simulink model "Good_1PF_Template_Copy"  (R2022b)
settings: Solver=FixedStepAuto  StartTime=0.0  StopTime=30  FixedStep=0.10  RelTol=1e-3
undefined symbols (not defined in the file): D1, D2, estimated_W_xu, initial_guess_belief_car2, num_particles, std_dev, W_xu_ranges, x0
settings Model: Creator=user  LastModifiedBy=user

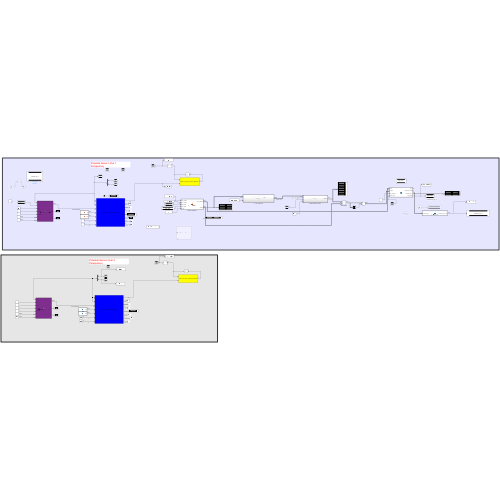
[thumbnail: Simulink's stored preview of the top-level diagram]
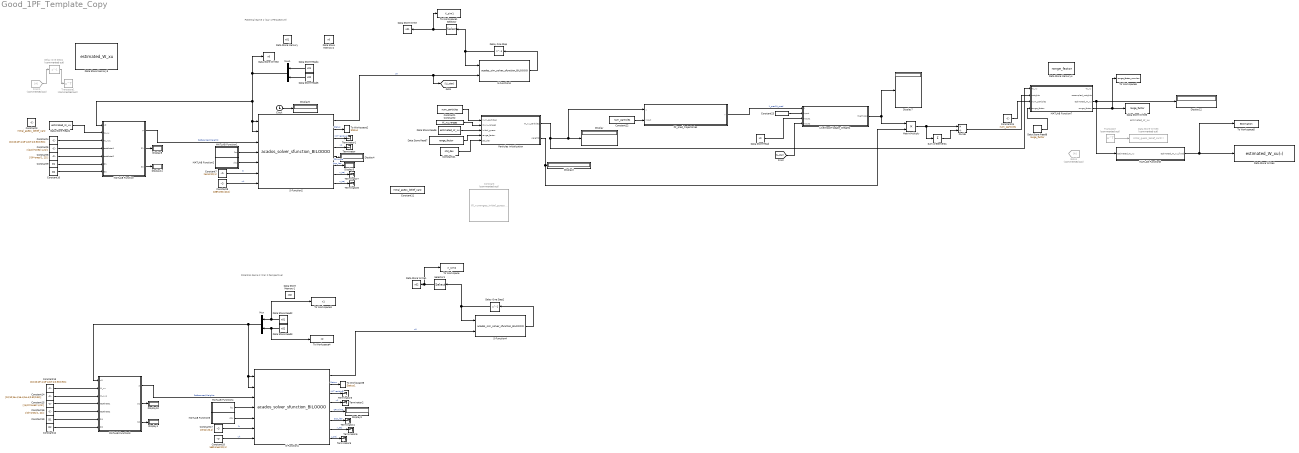
== system Good_1PF_Template_Copy ==
  note: estimated_W_xu
  note: Potential Game 1 (Car 1 Perspective)
  note: Potential Game 2 (Car 2 Perspective)
  Clock : Clock
  Constant : Constant  Commented=on  Value=W_xuranges_initial_guess...
  Constant{1,22..24} (4 alike) : Constant  Value=num_particles
  Constant10 : Constant  Value=D2
  Constant11 : Constant  Value=initial_guess_belief_car2
  Constant12 : Constant  Value=D2
  Constant13 : Constant  Value=[10;10;1e-4;1e-4;1e-4;0.50;0.50];
  Constant14 : Constant  Value=[10;10;1e-4;1e-4;1e-4;0.50;0.50];
  Constant15 : Constant  Value=[(pi/2)*ones(1,21)]
  Constant16 : Constant  Value=[(0)*ones(1, 21)]
  Constant17 : Constant  Value=zeros(20,1)
  Constant18 : Constant  Value=1e8*ones(20,1)
  Constant19 : Constant  Value=D1
  Constant2 : Constant  Value=W_xu_ranges
  Constant21 : Constant  Value=std_dev
  Constant3 : Constant  Value=initial_guess_belief_car2
  Constant4 : Constant  Value=[10;10;1e-4;1e-4;1e-4;0.50;0.50];
  Constant5 : Constant  Value=[(pi/2)*ones(1,21)]
  Constant6 : Constant  Value=[(0)*ones(1, 21)]
  Constant7 : Constant  Value=zeros(20,1)
  Constant8 : Constant  Value=1e8*ones(20,1)
  Constant9 : Constant  Value=D1
  Data Store Memory : DataStoreMemory  DataStoreName=x01  WriteAfterWriteMsg=warning  InitialValue=x01  ShowAdditionalParam=off
  Data Store Memory1 : DataStoreMemory  DataStoreName=x02  WriteAfterWriteMsg=warning  InitialValue=x02  ShowAdditionalParam=off
  Data Store Memory2 : DataStoreMemory  DataStoreName=x0  WriteAfterWriteMsg=warning  InitialValue=x0  ShareAcrossModelInstances=on  ShowAdditionalParam=off
  Data Store Memory3 : DataStoreMemory  DataStoreName=estimated_W_xu  WriteAfterWriteMsg=warning  InitialValue=initial_guess_belief_car2  ShowAdditionalParam=off
  Data Store Memory4 : DataStoreMemory  DataStoreName=range_factor  WriteAfterWriteMsg=warning  InitialValue=1  ShowAdditionalParam=off
  Data Store Read : DataStoreRead  DataStoreName=x0  IndexOptions=Index vector (dialog)  Indices=1  OutputSizes=1
  Data Store Read1 : DataStoreRead  DataStoreName=estimated_W_xu  IndexOptions=Index vector (dialog)  Indices=1  OutputSizes=1
  Data Store Read2 : DataStoreRead  DataStoreName=x01  IndexOptions=Index vector (dialog)  Indices=1  OutputSizes=1
  Data Store Read3 : DataStoreRead  DataStoreName=x02  IndexOptions=Index vector (dialog)  Indices=1  OutputSizes=1
  Data Store Read4 : DataStoreRead  DataStoreName=x01  IndexOptions=Index vector (dialog)  Indices=1  OutputSizes=1
  Data Store Read5 : DataStoreRead  DataStoreName=x02  IndexOptions=Index vector (dialog)  Indices=1  OutputSizes=1
  Data Store Read6 : DataStoreRead  DataStoreName=estimated_W_xu  IndexOptions=Index vector (dialog)  Indices=1  OutputSizes=1
  Data Store Read7 : DataStoreRead  DataStoreName=range_factor  IndexOptions=Index vector (dialog)  Indices=1  OutputSizes=1
  Data Store Read8 : DataStoreRead  DataStoreName=range_factor  IndexOptions=Index vector (dialog)  Indices=1  OutputSizes=1
  Data Store Write : DataStoreWrite  DataStoreName=x01  DataStoreElements=x01  IndexOptions=Index vector (dialog)  Indices=1  OutputSizes=1
  Data Store Write1 : DataStoreWrite  DataStoreName=x02  IndexOptions=Index vector (dialog)  Indices=1  OutputSizes=1
  Data Store Write2 : DataStoreWrite  DataStoreName=x0  IndexOptions=Index vector (dialog)  Indices=1  OutputSizes=1
  Data Store Write3 : DataStoreWrite  Commented=on  DataStoreName=initial_guess_belief_car2  DataStoreElements=initial_guess_belief_car2(:)  IndexOptions=Index vector (dialog)  Indices=1  OutputSizes=1
  Data Store Write4 : DataStoreWrite  DataStoreName=estimated_W_xu  DataStoreElements=estimated_W_xu(:)  IndexOptions=Index vector (dialog)  Indices=1  OutputSizes=1
  Data Store Write5 : DataStoreWrite  DataStoreName=range_factor  IndexOptions=Index vector (dialog)  Indices=1  OutputSizes=1
  Delay One Step : Delay  DelayLength=1  InitialCondition=x0
  Delay One Step1 : Delay  Commented=on  DelayLength=1  InitialCondition=initial_guess_belief_car2'
  Delay One Step2 : Delay  DelayLength=1  InitialCondition=x0
  Display{,1..8,10..12} (12 alike) : Display
  Divide : Product  Inputs=*/
  From1 : From  Commented=on
  Goto1 : Goto  Commented=on
  Likelihood+Ipdate_Weights : Subsystem  TreatAsAtomicUnit=on
  MATLAB Function : MATLAB Function  TreatAsAtomicUnit=on
  MATLAB Function1 : MATLAB Function  TreatAsAtomicUnit=on
  MATLAB Function2 : MATLAB Function  TreatAsAtomicUnit=on
  MATLAB Function3 : MATLAB Function  TreatAsAtomicUnit=on
  MATLAB Function4 : MATLAB Function  TreatAsAtomicUnit=on
  MATLAB Function5 : MATLAB Function  TreatAsAtomicUnit=on
  MATLAB Function7 : MATLAB Function  TreatAsAtomicUnit=on
  MATLAB Function8 : MATLAB Function  TreatAsAtomicUnit=on
  MatrixMultiply : Product
  Mux : Mux  Inputs=2
  Mux1 : Mux  Inputs=2
  PF_pred_trajectories : Subsystem  TreatAsAtomicUnit=on
  Particles initialization : MATLAB Function  TreatAsAtomicUnit=on
  S-Function1 : S-Function  FunctionName=acados_solver_sfunction_BILOOOO  SFunctionDeploymentMode=off  EnableBusSupport=off
  S-Function2 : S-Function  FunctionName=acados_solver_sfunction_BILOOOO  SFunctionDeploymentMode=off  EnableBusSupport=off
  S-Function3 : S-Function  FunctionName=acados_sim_solver_sfunction_BILOOOO  SFunctionDeploymentMode=off  EnableBusSupport=off
  S-Function4 : S-Function  FunctionName=acados_sim_solver_sfunction_BILOOOO  SFunctionDeploymentMode=off  EnableBusSupport=off
  Selector : Selector  InputPortWidth=10  IndexOptions=Index vector (dialog)  Indices=[1:5]  OutputSizes=1
  Selector1 : Selector  InputPortWidth=10  IndexOptions=Index vector (dialog)  Indices=[6:10]  OutputSizes=1
  Sum of Elements : Sum  Inputs=+
  Terminator{,1..8} (9 alike) : Terminator
  To Workspace : ToWorkspace  VariableName=X_sim2  SaveFormat=Structure With Time  SampleTime=-1
  To Workspace1 : ToWorkspace  VariableName=X_sim1  SaveFormat=Structure With Time  SampleTime=-1
  To Workspace2 : ToWorkspace  VariableName=Status  SampleTime=-1
      settings: Save2DSignal=2-D array (concatenate along first dimension)
  To Workspace3 : ToWorkspace  VariableName=x1  SaveFormat=Structure  SampleTime=-1
  To Workspace4 : ToWorkspace  VariableName=x2  SaveFormat=Structure  SampleTime=-1
  To Workspace5 : ToWorkspace  VariableName=Estimation  SampleTime=-1
      settings: Save2DSignal=2-D array (concatenate along first dimension)
  To Workspace6 : ToWorkspace  VariableName=range_factor_monitor  SampleTime=-1
      settings: Save2DSignal=2-D array (concatenate along first dimension)
  To Workspace8 : ToWorkspace  VariableName=Status1  SampleTime=-1
      settings: Save2DSignal=2-D array (concatenate along first dimension)
  Transpose : Math  Commented=on  Operator=transpose
  Transpose1 : Math  Commented=on  Operator=transpose
  wires:
  Constant14/1 -> MATLAB Function3/3(W_xu1)
  Mux1/1 -> Data Store Write2/1, S-Function2/2, S-Function2/1, MATLAB Function/1(x0)
  Data Store Read5/1 -> Mux1/2
  S-Function4/1 -> Delay One Step2/1
  Constant19/1 -> MATLAB Function3/6(D1)
  Constant15/1 -> MATLAB Function3/4(testtheta1)
  Constant7/1 -> S-Function2/6  "lh"
  MATLAB Function1/1(lbu) -> S-Function2/4
  MATLAB Function/2(S1) -> Display8/1
  MATLAB Function/1(p) -> S-Function2/3  "References|Weights"
  S-Function2/4 -> Terminator/1  "x1"
  Data Store Read3/1 -> To Workspace4/1, Mux/2
  MATLAB Function3/3(S2) -> Display1/1
  S-Function1/7 -> Terminator6/1  "x_traj"
  S-Function2/3 -> Terminator1/1  "KKT residual"
  MATLAB Function4/1(lbu) -> S-Function1/4
  Delay One Step/1 -> Selector/1, S-Function3/1
  Constant13/1 -> MATLAB Function3/2(W_xu)
  Constant17/1 -> S-Function1/6  "lh"
  S-Function3/1 -> Delay One Step/1
  Constant8/1 -> S-Function2/7  "uh"
  MATLAB Function/3(S2) -> Display11/1
  Delay One Step2/1 -> Selector1/1, S-Function4/1
  S-Function2/2 -> To Workspace2/1  "Status"
  S-Function1/2 -> To Workspace8/1  "Status"
  MATLAB Function3/1(p) -> S-Function1/3  "References|Weights"
  MATLAB Function5/1(ubu) -> S-Function1/5
  S-Function1/3 -> Terminator3/1  "KKT residual"
  Clock/1 -> Display6/1
  Constant10/1 -> MATLAB Function/7(D2)
  S-Function2/8 -> Terminator8/1  "u_traj"
  S-Function1/5 -> Display3/1  "CPU time"
  S-Function1/4 -> Terminator2/1  "x1"
  Constant4/1 -> MATLAB Function/3(W_xu1)
  Constant16/1 -> MATLAB Function3/5(testtheta2)
  MATLAB Function2/1(ubu) -> S-Function2/5
  Mux/1 -> S-Function1/2, S-Function1/1, MATLAB Function3/1(x0)
  Data Store Read4/1 -> Mux1/1
  S-Function1/6 -> Terminator4/1  "Sqp_iter"
  Constant6/1 -> MATLAB Function/5(testtheta2)
  S-Function1/1 -> S-Function4/2  "u0"
  S-Function2/6 -> Display5/1  "Sqp_iter"
  S-Function2/1 -> [U_star], S-Function3/2  "u0"
  MATLAB Function3/2(S1) -> Display10/1
  S-Function1/8 -> Terminator5/1  "u_traj"
  Constant5/1 -> MATLAB Function/4(testtheta1)
  Selector/1 -> To Workspace1/1, Data Store Write/1
  Selector1/1 -> To Workspace/1, Data Store Write1/1
  S-Function2/5 -> Display4/1  "CPU time"
  Constant9/1 -> MATLAB Function/6(D1)
  S-Function2/7 -> Terminator7/1  "x_traj"
  Data Store Read2/1 -> To Workspace3/1, Mux/1
  Constant12/1 -> MATLAB Function3/7(D2)
  Constant18/1 -> S-Function1/7  "uh"
  Constant1/1 -> Particles initialization/1(num_particles)
  Data Store Read7/1 -> Particles initialization/4(range_factor)
  Constant2/1 -> Particles initialization/2(W_xu_ranges)
  Constant21/1 -> Particles initialization/5(std_dev)
  Particles initialization/1(W_xu_particles) -> PF_pred_trajectories/1(y), Display/1, MATLAB Function7/1("W_xu ")
  Particles initialization/2(weights) -> MatrixMultiply/2, Display2/1
  Constant22/1 -> PF_pred_trajectories/2(Input)
  PF_pred_trajectories/1(Y) -> Likelihood+Ipdate_Weights/1(Y)  "X_pred|U_pred"
  Constant23/1 -> Likelihood+Ipdate_Weights/2(Input)
  Data Store Read/1 -> Likelihood+Ipdate_Weights/3(Input1)
  [U_star] -> Likelihood+Ipdate_Weights/4(Input2)
  Likelihood+Ipdate_Weights/1(likelihood) -> MatrixMultiply/1, Display7/1
  MatrixMultiply/1 -> Sum of Elements/1, Divide/1
  Sum of Elements/1 -> Divide/2
  Divide/1 -> MATLAB Function7/2(weights)
  Constant24/1 -> MATLAB Function7/3(num_particles)
  MATLAB Function7/3(estimated_W_xu) -> MATLAB Function8/1(estimated_W_xu), Display12/1
  Transpose/1 -> Data Store Write3/1
  From1/1 -> Delay One Step1/1
  Delay One Step1/1 -> Transpose1/1
  Data Store Read1/1 -> MATLAB Function/2(W_xu)
  MATLAB Function8/1(estimated_W_xu_fixed) -> To Workspace5/1, Data Store Write4/1
  Data Store Read6/1 -> Particles initialization/3(initial_guess)
  MATLAB Function7/4(range_factor) -> To Workspace6/1, Data Store Write5/1
  Data Store Read8/1 -> MATLAB Function7/4("range_factor ")

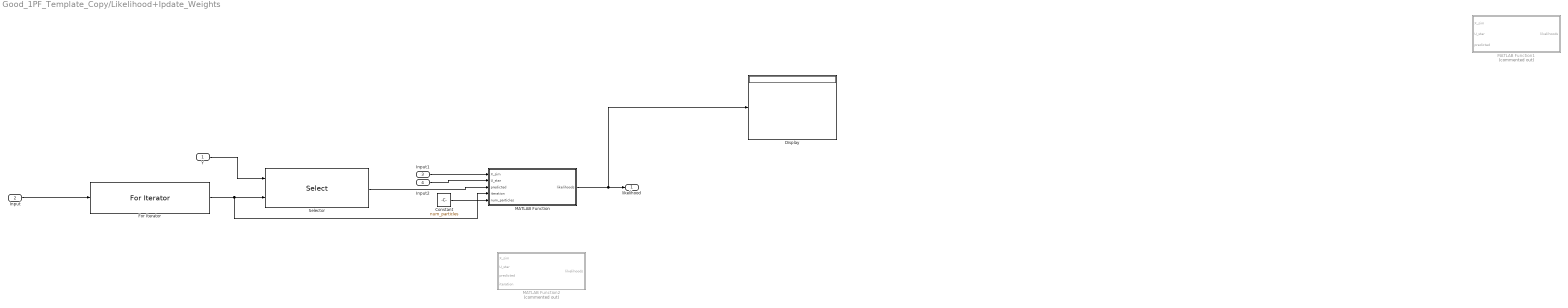
== system Good_1PF_Template_Copy/Likelihood+Ipdate_Weights ==
  Y : Inport
  Input : Inport  Port=2
  Input1 : Inport  Port=3
  Input2 : Inport  Port=4
  Constant : Constant  Value=num_particles
  Display : Display
  For Iterator : ForIterator  IterationSource=external
  MATLAB Function : MATLAB Function  TreatAsAtomicUnit=on
  MATLAB Function1 : MATLAB Function  Commented=on  TreatAsAtomicUnit=on
  MATLAB Function2 : MATLAB Function  Commented=on  TreatAsAtomicUnit=on
  Selector : Selector  NumberOfDimensions=2  IndexOptions=Select all,Index vector (port)  Indices=[1 3],1  OutputSizes=1,1  RuntimeRangeChecks=on
  likelihood : Outport
  wires:
  Input/1 -> For Iterator/1
  For Iterator/1 -> MATLAB Function/4(iteration), Selector/2
  Y/1 -> Selector/1
  Selector/1 -> MATLAB Function/3(predicted)
  Input1/1 -> MATLAB Function/1(X_sim)
  Input2/1 -> MATLAB Function/2(U_star)
  MATLAB Function/1(likelihoods) -> Display/1, likelihood/1
  Constant/1 -> MATLAB Function/5(num_particles)

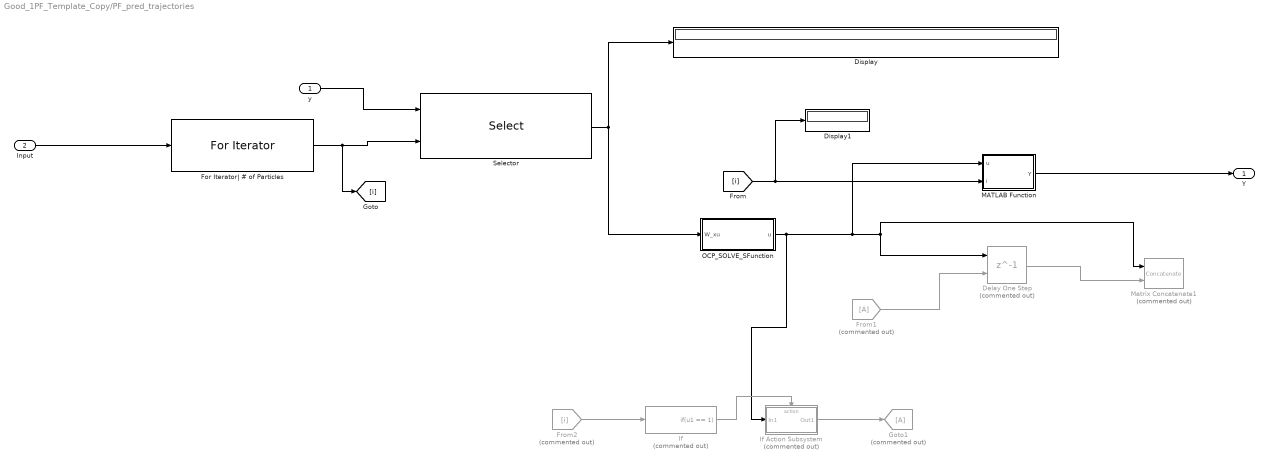
== system Good_1PF_Template_Copy/PF_pred_trajectories ==
  y : Inport
  Input : Inport  Port=2
  Delay One Step : Delay  Commented=on  DelayLength=1  InitialConditionSource=Input port
      settings: InputPortMap=u0,p4
  Display : Display
  Display1 : Display
  For Iterator| # of Particles : ForIterator  IterationSource=external  IterationLimit=num_particles
  From1 : From  Commented=on
  From2 : From  Commented=on  GotoTag=i
  Goto1 : Goto  Commented=on
  If : If  Commented=on  IfExpression=u1 == 1  ShowElse=off
  If Action Subsystem : Subsystem  Commented=on  TreatAsAtomicUnit=on
  MATLAB Function : MATLAB Function  TreatAsAtomicUnit=on
  Matrix Concatenate1 : Concatenate  Commented=on  Mode=Multidimensional array  ConcatenateDimension=2
  OCP_SOLVE_SFunction : Subsystem
  Selector : Selector  NumberOfDimensions=2  IndexOptions=Index vector (port),Select all  Indices=[1 3],1  OutputSizes=1,1  RuntimeRangeChecks=on
  Y : Outport
  wires:
  Input/1 -> For Iterator| # of Particles/1
  For Iterator| # of Particles/1 -> [i], Selector/2
  y/1 -> Selector/1
  Selector/1 -> OCP_SOLVE_SFunction/1(W_xu), Display/1
  OCP_SOLVE_SFunction/1(u) -> MATLAB Function/1(u), Delay One Step/1, Matrix Concatenate1/1, If Action Subsystem/1(In1)
  If Action Subsystem/1(Out1) -> Goto1/1
  From1/1 -> Delay One Step/2
  Delay One Step/1 -> Matrix Concatenate1/2
  From2/1 -> If/1
  If/1 -> If Action Subsystem/Action
  [i] -> Display1/1, MATLAB Function/2(i)
  MATLAB Function/1(Y) -> Y/1

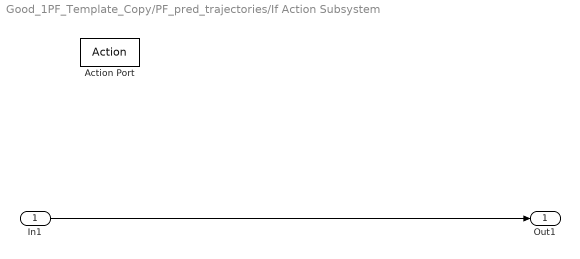
== system Good_1PF_Template_Copy/PF_pred_trajectories/If Action Subsystem ==
  In1 : Inport
  Action Port : ActionPort  ActionPortLabel=if(u1 == 1)
  Out1 : Outport
  wires:
  In1/1 -> Out1/1

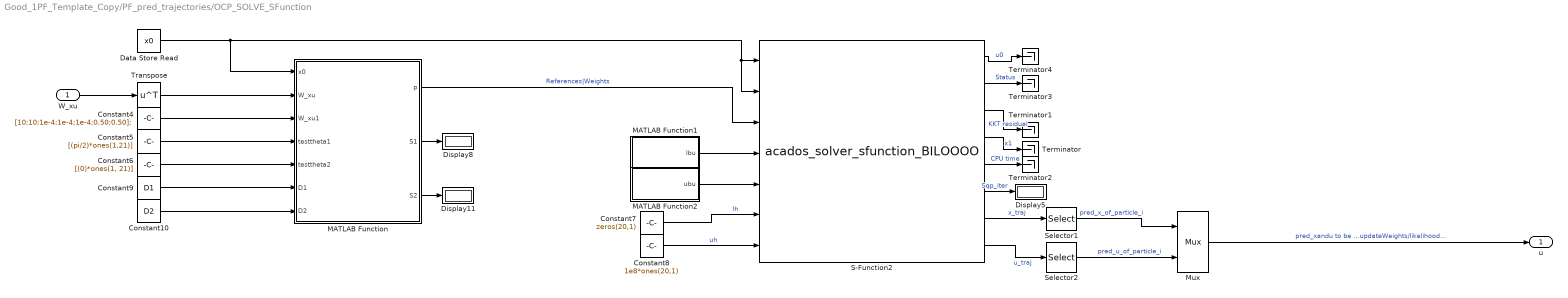
== system Good_1PF_Template_Copy/PF_pred_trajectories/OCP_SOLVE_SFunction ==
  W_xu : Inport
  Constant10 : Constant  Value=D2
  Constant4 : Constant  Value=[10;10;1e-4;1e-4;1e-4;0.50;0.50];
  Constant5 : Constant  Value=[(pi/2)*ones(1,21)]
  Constant6 : Constant  Value=[(0)*ones(1, 21)]
  Constant7 : Constant  Value=zeros(20,1)
  Constant8 : Constant  Value=1e8*ones(20,1)
  Constant9 : Constant  Value=D1
  Data Store Read : DataStoreRead  DataStoreName=x0  IndexOptions=Index vector (dialog)  Indices=1  OutputSizes=1
  Display11 : Display
  Display5 : Display
  Display8 : Display
  MATLAB Function : MATLAB Function  TreatAsAtomicUnit=on
  MATLAB Function1 : MATLAB Function  TreatAsAtomicUnit=on
  MATLAB Function2 : MATLAB Function  TreatAsAtomicUnit=on
  Mux : Mux  Inputs=2
  S-Function2 : S-Function  FunctionName=acados_solver_sfunction_BILOOOO  SFunctionDeploymentMode=off  EnableBusSupport=off
  Selector1 : Selector  InputPortWidth=210  IndexOptions=Index vector (dialog)  Indices=[11:20]  OutputSizes=1
  Selector2 : Selector  InputPortWidth=80  IndexOptions=Index vector (dialog)  Indices=[1:4]  OutputSizes=1
  Terminator{,1..4} (5 alike) : Terminator
  Transpose : Math  Operator=transpose
  u : Outport
  wires:
  MATLAB Function1/1(lbu) -> S-Function2/4
  Data Store Read/1 -> S-Function2/2, S-Function2/1, MATLAB Function/1(x0)
  S-Function2/3 -> Terminator1/1  "KKT residual"
  Constant6/1 -> MATLAB Function/5(testtheta2)
  MATLAB Function/2(S1) -> Display8/1
  S-Function2/7 -> Selector1/1  "x_traj"
  Constant4/1 -> MATLAB Function/3(W_xu1)
  MATLAB Function/1(p) -> S-Function2/3  "References|Weights"
  S-Function2/6 -> Display5/1  "Sqp_iter"
  MATLAB Function2/1(ubu) -> S-Function2/5
  Constant8/1 -> S-Function2/7  "uh"
  S-Function2/5 -> Terminator2/1  "CPU time"
  Constant5/1 -> MATLAB Function/4(testtheta1)
  MATLAB Function/3(S2) -> Display11/1
  Constant9/1 -> MATLAB Function/6(D1)
  S-Function2/4 -> Terminator/1  "x1"
  S-Function2/2 -> Terminator3/1  "Status"
  Constant10/1 -> MATLAB Function/7(D2)
  S-Function2/8 -> Selector2/1  "u_traj"
  Constant7/1 -> S-Function2/6  "lh"
  S-Function2/1 -> Terminator4/1  "u0"
  Selector1/1 -> Mux/1  "pred_x_of_particle_i"
  Selector2/1 -> Mux/2  "pred_u_of_particle_i"
  Mux/1 -> u/1  "pred_xandu to be fed into the updateWeights/likelihood..."
  W_xu/1 -> Transpose/1
  Transpose/1 -> MATLAB Function/2(W_xu)

== matlab function Good_1PF_Template_Copy/Particles initialization ==
  data: num_particles input; W_xu_particles output size=[num_particles, 7] [..100000]; W_xu_ranges input; initial_guess input; range_factor input; std_dev input; weights output size=[num_particles,1] [-1..10]
function [W_xu_particles,weights] = initializeParticles1(num_particles, W_xu_ranges,initial_guess,range_factor,std_dev)
    num_ranges = size(W_xu_ranges, 1);  % Number of parameters
    W_xu_particles = zeros(num_particles, num_ranges);

    std_dev=std_dev*range_factor;

    
    for i = 1:num_ranges
        % Define the mean and standard deviation for the Gaussian distribution for parameter i
        mean_value = initial_guess(i)    % Mean for the Gaussian distribution
        std_deviation = std_dev(i);          % Standard deviation for the Gaussian distribution

        % Generate random particles from a Gaussian distribution
        W_xu_particles(:, i) = mean_value + std_deviation * randn(num_particles, 1)
        
        % Clip values to be within the specified range
        W_xu_particles(:, i) = max(W_xu_ranges(i, 1), min(W_xu_ranges(i, 2), W_xu_particles(:, i)));
    end
    %%% make the x and y the same since we have that knowledge (testing this)
    W_xu_particles(:,2)=W_xu_particles(:,1);
    %%%
    
    % Initialize weights uniformly
    weights = ones(num_particles, 1) / num_particles;
%     
%     particles.W_xu = W_xu_particles;
%     particles.weights = weights;
end

== matlab function Good_1PF_Template_Copy/Likelihood+Ipdate_Weights/MATLAB Function ==
  data: X_sim input; U_star input; likelihoods output size=[num_particles,1]; predicted input; iteration input; num_particles input
function likelihoods = computeLikelihood(X_sim, U_star, predicted, iteration, num_particles)
    % Inputs:
    % X_sim: Actual state trajectory (Nx1)
    % U_star: Actual control inputs (Nu x 1)
    % predicted: A matrix containing both predicted trajectory and control inputs (14 x num_particles)
    % iteration: Current iteration index from the for iterator
    % num_particles: Number of particles used

%     % Initialize likelihood_storage to zeros at the start of each PF
%     persistent likelihood_storage;
% 
%     % Initialize on the first call or reset after each PF
%     if isempty(likelihood_storage) || length(likelihood_storage) ~= num_particles
%         likelihood_storage = zeros(num_particles, 1); % Initialize as zeros
%     end
    likelihood_storage=zeros(num_particles,1);

    % Parameters
    std_state = [0.1; 0.1; 0.01; 0.05; 0.02];  % For (x, y, theta, velocity, steering)
    std_control = [0.1; 0.01];  % For (acceleration, steering rate)

    % Extract predicted trajectory and control inputs for the current particle
    predicted_trajectory = predicted(1:10); % First 10 elements for states
    predicted_control = predicted(11:14);   % Last 4 elements for control inputs

    % Compute the deviation between predicted and observed state trajectory
    state_deviation = X_sim - predicted_trajectory;

    % Compute the deviation between predicted and observed control inputs
    control_deviation = U_star - predicted_control;

    % Compute weighted errors
    weighted_state_error = sum(state_deviation.^2);
    weighted_control_error = sum(control_deviation.^2);

    % Combine state and control errors
    total_error = weighted_state_error + weighted_control_error;
    scaling_factor = 10 / (max(std(state_deviation(:)), std(control_deviation(:))) + 1e-5); % Adjust as necessary

    % Compute likelihood
    likelihood = exp(-0.5 * scaling_factor * total_error);
    likelihood = max(likelihood, 1e-30); % Ensure likelihood is within reasonable range

    % Update the likelihood storage for the current iteration
    likelihood_storage(iteration) = likelihood;

    % Output the accumulated likelihoods
    likelihoods = likelihood_storage; % Output the accumulated likelihoods
end

== matlab function Good_1PF_Template_Copy/Likelihood+Ipdate_Weights/MATLAB Function1 ==
  data: X_sim input; U_star input; likelihoods output; predicted input
% function [likelihood, total_error] = computeLikelihood(X_sim, predicted_trajectory, U_star)
%     % Extract state and control inputs
%     nx = 10;  % Number of state variables
%     nu = 4;   % Number of control inputs
% 
%     % Assuming predicted_trajectory is a 14x1 vector
%     predicted_states = predicted_trajectory(1:nx); % First 10 elements for states
%     predicted_control = predicted_trajectory(nx+1:end); % Last 4 elements for controls
% 
%     std_state = [0.1; 0.1; 0.01; 0.05; 0.02];  % For (x, y, theta, velocity, steering)
%     std_control = [0.1; 0.01];  % For (acceleration, steering rate)
% 
%     % Compute the deviation between predicted and observed state trajectory
%     state_deviation = X_sim - predicted_states;
% 
%     % Compute the deviation between predicted and observed control inputs
%     control_deviation = U_star - predicted_control;
% 
%     % Assuming state variables are weighted
%     importance_state_weights = [1, 1, 1e-5, 1e-5, 1e-5]; % Weights for state variables
%     importance_control_weights = [1, 1];                 % Weights for control inputs
%     
%     % Noise-based weights
%     noise_state_weights = 1 ./ (2 * std_state.^2);  % State noise
%     noise_control_weights = 2 * std_control.^2;  % Control noise
% 
%     combined_state_weights = importance_state_weights ./ (1 + noise_state_weights);
%     normalized_weights_state = combined_state_weights / sum(combined_state_weights);
% 
%     combined_control_weights = importance_control_weights .* (1 ./ (1 + noise_control_weights));
%     normalized_weights_control = combined_control_weights / sum(combined_control_weights);
% 
%     % Compute weighted state and control errors
%     weighted_state_error = sum((normalized_weights_state' .* state_deviation).^2, 1);
%     weighted_control_error = sum((normalized_weights_control' .* control_deviation).^2, 1);
% 
%     % Combine state and control errors
%     total_error = sum(weighted_state_error) + sum(weighted_control_error);
% 
%     norm_state_error = state_deviation ./ (std(state_deviation(:)) + 1e-5);
%     norm_control_error = control_deviation ./ (std(control_deviation(:)) + 1e-5);
%     
%     scaling_factor = 10 * 1 / (max(std(norm_state_error), std(norm_control_error)) + 1e-5);
% 
%     % Compute likelihood
%     likelihood = exp(-0.5 * scaling_factor * total_error);
%     likelihood = max(likelihood, 1e-30); % Ensure likelihood is within a reasonable range
% end

function likelihoods = computeLikelihoods(X_sim, U_star, predicted)
    % Inputs:
    % X_sim: Actual state trajectory (Nx1)
    % U_star: Actual control inputs (Nu x 1)
    % predicted: A matrix containing both predicted trajectory and control inputs (14 x num_particles)

    % Parameters
    num_particles = size(predicted, 2); % Number of particles
    likelihoods = zeros(num_particles, 1); % Preallocate array for likelihoods

    std_state = [0.1; 0.1; 0.01; 0.05; 0.02];  % For (x, y, theta, velocity, steering)
    std_control = [0.1; 0.01];  % For (acceleration, steering rate)

    % Loop through each particle
    for i = 1:num_particles
        % Extract predicted trajectory and control inputs for the current particle
        predicted_trajectory = predicted(1:10, i); % First 10 elements for states
        predicted_control = predicted(11:14, i);   % Last 4 elements for control inputs

        % Compute the deviation between predicted and observed state trajectory
        state_deviation = X_sim - predicted_trajectory;

        % Compute the deviation between predicted and observed control inputs
        control_deviation = U_star - predicted_control;

        % Compute weighted errors (adjust according to your weighting scheme)
        weighted_state_error = sum(state_deviation.^2);
        weighted_control_error = sum(control_deviation.^2);

        % Combine state and control errors
        total_error = weighted_state_error + weighted_control_error;
        scaling_factor = 10 / (max(std(state_deviation(:)), std(control_deviation(:))) + 1e-5); % Adjust as necessary

        % Compute likelihood
        likelihood = exp(-0.5 * scaling_factor * total_error);
        likelihood = max(likelihood, 1e-30); % Ensure likelihood is within reasonable range

        % Store the likelihood for this particle
        likelihoods(i) = likelihood;
    end
end

== matlab function Good_1PF_Template_Copy/MATLAB Function7 ==
  data: W_xu input; W_xu output; resampled_weights output size=[num_particles,1]; weights input; num_particles input; estimated_W_xu output size=[1,7]; range_factor output; range_factor input
function [W_xu, resampled_weights,estimated_W_xu,range_factor] = resampleParticles(W_xu, weights,num_particles,range_factor)
    % Inputs:
    % - W_xu: Matrix of particle states and weights (num_particles x 7)
    % - weights: Current particle weights (num_particles x 1)
    %
    % Outputs:
    % - W_xu: Resampled particle matrix (num_particles x 7)
    % - resampled_weights: Uniform weights after resampling (num_particles x 1)

  
    % Normalize weights
%     weights = weights / sum(weights);

    % Resample particle indices based on the updated weights
    estimated_W_xu=zeros(1,7);
    resampled_weights=zeros(num_particles,1);

    resample_indices = randsample(1:num_particles, num_particles, true, weights);

    % Resample particles using the indices
    W_xu = W_xu(resample_indices, :); 

    % Reset weights to uniform distribution after resampling
    resampled_weights = ones(num_particles, 1) / num_particles;

    % Return the updated W_xu, pre-resample weights, and resampled weights


     % Element-wise multiplication of W_xu by weights
    weighted_W_xu = W_xu .* resampled_weights;

    % Sum the weighted values across the particles (i.e., summing along rows)
    estimated_W_xu = sum(weighted_W_xu, 1); % Output will be 1x7
    range_factor=range_factor*0.995;
    range_factor=max(0.10,range_factor);
end

== matlab function Good_1PF_Template_Copy/MATLAB Function8 ==
  data: estimated_W_xu input; estimated_W_xu_fixed output
function estimated_W_xu_fixed = padVariableSize(estimated_W_xu)
    %#codegen
    % Declare fixed-size array
    estimated_W_xu_fixed = zeros(1, 7);
    
    % Fill the array with the variable-size signal
    estimated_W_xu_fixed(1:numel(estimated_W_xu)) = estimated_W_xu;
end

== matlab function Good_1PF_Template_Copy/Likelihood+Ipdate_Weights/MATLAB Function2 ==
  data: X_sim input; U_star input; likelihoods output size=[num_particles,1]; predicted input; iteration input
function likelihoods = computeLikelihood(X_sim, U_star, predicted, iteration)
    % Inputs:
    % X_sim: Actual state trajectory (Nx1)
    % U_star: Actual control inputs (Nu x 1)
    % predicted: A matrix containing both predicted trajectory and control inputs (14 x num_particles)
    % iteration: Current iteration index from the for iterator
%     likelihoods = zeros(num_particles,1);

    % Persistent variable to store likelihoods
    persistent likelihood_storage;

    if isempty(likelihood_storage) % Initialize on the first call
        likelihood_storage = []; % Initialize as an empty array
    end

    % Parameters
    std_state = [0.1; 0.1; 0.01; 0.05; 0.02];  % For (x, y, theta, velocity, steering)
    std_control = [0.1; 0.01];  % For (acceleration, steering rate)

    % Extract predicted trajectory and control inputs for the current particle
    predicted_trajectory = predicted(1:10, 1); % First 10 elements for states
    predicted_control = predicted(11:14, 1);   % Last 4 elements for control inputs

    % Compute the deviation between predicted and observed state trajectory
    state_deviation = X_sim - predicted_trajectory;

    % Compute the deviation between predicted and observed control inputs
    control_deviation = U_star - predicted_control;

    % Compute weighted errors
    weighted_state_error = sum(state_deviation.^2);
    weighted_control_error = sum(control_deviation.^2);

    % Combine state and control errors
    total_error = weighted_state_error + weighted_control_error;
    scaling_factor = 10 / (max(std(state_deviation(:)), std(control_deviation(:))) + 1e-5); % Adjust as necessary

    % Compute likelihood
    likelihood = exp(-0.5 * scaling_factor * total_error);
    likelihood = max(likelihood, 1e-30); % Ensure likelihood is within reasonable range

    % Store the likelihood
    likelihood_storage = [likelihood_storage; likelihood]; % Append to storage

    % Output the accumulated likelihoods
    likelihoods = likelihood_storage; % Output the accumulated likelihoods
end

== matlab function Good_1PF_Template_Copy/MATLAB Function1 ==
  data: lbu output
function lbu = LBU
% Define lower bounds for control inputs
lbu_control = [-11.5; -1; -11.5; -1]; % Control inputs

% Determine how many times to repeat the control bounds
num_repeats = ceil(80 / length(lbu_control)); % Calculate how many times to repeat
lbu = repmat(lbu_control, num_repeats, 1); % Repeat to create a long enough array
lbu = lbu(1:80); % Truncate to exactly 80 elements

% Check size
assert(length(lbu) == 80, 'Lower bounds array must have 80 elements.');

end

== matlab function Good_1PF_Template_Copy/MATLAB Function ==
  data: x0 input; p output; W_xu input; W_xu1 input; testtheta1 input; testtheta2 input; D1 input; D2 input; S1 output; S2 output
function [p, S1, S2] = OCP_prepare_parameters(x0, W_xu, W_xu1, testtheta1, testtheta2, D1, D2)
    nx = length(x0);
    nu = 4;
    ocp_N = 20; % Number of prediction steps
    % Initialize the parameter array
    p = zeros(504, 1); % 504 elements as per your structure

    % Prepare reference points
    current_state1 = x0(1:2); % Use the updated x0 for car 1
    current_state2 = x0(6:7); % Use the updated x0 for car 2
    
    closest_idx1 = findClosestPoint(current_state1, D1);
    closest_idx2 = findClosestPoint(current_state2, D2);
    
    % Reference points for car 1
    if closest_idx1 + ocp_N <= size(D1, 2)
        reference_points1 = D1(:, closest_idx1:closest_idx1 + ocp_N);
    else
        remaining_points1 = size(D1, 2) - closest_idx1 + 1;
        reference_points1 = D1(:, closest_idx1:end);
        additional_points1 = (ocp_N + 1) - remaining_points1;

        last_x1 = D1(1, end);
        last_y1 = D1(2, end);
        new_x1 = last_x1 - (1:additional_points1) * 0.1; % Assuming 0.1m per step
        new_y1 = last_y1 * ones(1, additional_points1);

        extended_points1 = [new_x1; new_y1];
        reference_points1 = [reference_points1, extended_points1];
    end
    
    % Reference points for car 2
    if closest_idx2 + ocp_N <= size(D2, 2)
        reference_points2 = D2(:, closest_idx2:closest_idx2 + ocp_N);
    else
        remaining_points2 = size(D2, 2) - closest_idx2 + 1;
        reference_points2 = D2(:, closest_idx2:end);
        additional_points2 = (ocp_N + 1) - remaining_points2;

        last_x2 = D2(1, end);
        last_y2 = D2(2, end);
        new_x2 = last_x2 + (1:additional_points2) * 0.1; % Assuming 0.1m per step
        new_y2 = last_y2 * ones(1, additional_points2);

        extended_points2 = [new_x2; new_y2];
        reference_points2 = [reference_points2, extended_points2];
    end

    % Create x_traj_init with the specified structure
    x_traj_init = [
        reference_points1; % x1, y1, ...
        testtheta1';       % theta1
        zeros(1, ocp_N + 1); % v1
        zeros(1, ocp_N + 1); % s1
        reference_points2; % x2, y2, ...
        testtheta2';       % theta2
        zeros(1, ocp_N + 1); % v2
        zeros(1, ocp_N + 1)  % s2
    ];

    % Check sizes
    S1 = size(x_traj_init, 1); % Number of rows
    S2 = size(x_traj_init, 2); % Number of columns

%     % Ensure that x_traj_init has enough rows
%     if S1 < 20
%         error('x_traj_init does not have enough rows. Current size: %d', S1);
%     end

    % Fill the parameter array with references and weights
    for jj = 0:ocp_N
        % Fill references for the first car
        p((jj) * (10 + 14) + 1:(jj) * (10 + 14) + 5) = x_traj_init(1:5, jj + 1); % Ref for car 1
        
        % Fill references for the second car
        p((jj) * (10 + 14) + 6:(jj) * (10 + 14) + 10) = x_traj_init(6:10, jj + 1); % Ref for car 2
        
        % Fill weights for the first car
        p((jj) * (10 + 14) + 11:(jj) * (10 + 14) + 15) = W_xu1(1:5); % Weights for car 1
        
        % Fill weights for the second car
        p((jj) * (10 + 14) + 16:(jj) * (10 + 14) + 20) = W_xu(1:5); % Weights for car 2
        
        % Fill weights for the control inputs
        p((jj) * (10 + 14) + 21:(jj) * (10 + 14) + 24) = [W_xu(6:7);W_xu1(6:7)]; % Control input weights (4 elements)
    end

    % Check if the size of p is correct
    assert(length(p) == 504, 'Parameter array must have 504 elements.');

    % Output parameter array
end

== matlab function Good_1PF_Template_Copy/MATLAB Function2 ==
  data: ubu output
function ubu = UBU
% Define lower bounds for control inputs
ubu_control = [+11.5; 1; 11.5; 1]; % Control inputs

% Determine how many times to repeat the control bounds
num_repeats = ceil(80 / length(ubu_control)); % Calculate how many times to repeat
ubu = repmat(ubu_control, num_repeats, 1); % Repeat to create a long enough array
ubu = ubu(1:80); % Truncate to exactly 80 elements

% Check size
assert(length(ubu) == 80, 'Lower bounds array must have 80 elements.');

end

== matlab function Good_1PF_Template_Copy/MATLAB Function3 ==
  data: x0 input; p output; W_xu input; W_xu1 input; testtheta1 input; testtheta2 input; D1 input; D2 input; S1 output; S2 output
function [p, S1, S2] = OCP_prepare_parameters(x0, W_xu, W_xu1, testtheta1, testtheta2, D1, D2)
    nx = length(x0);
    nu = 4;
    ocp_N = 20; % Number of prediction steps
    % Initialize the parameter array
    p = zeros(504, 1); % 504 elements as per your structure

    % Prepare reference points
    current_state1 = x0(1:2); % Use the updated x0 for car 1
    current_state2 = x0(6:7); % Use the updated x0 for car 2
    
    closest_idx1 = findClosestPoint(current_state1, D1);
    closest_idx2 = findClosestPoint(current_state2, D2);
    
    % Reference points for car 1
    if closest_idx1 + ocp_N <= size(D1, 2)
        reference_points1 = D1(:, closest_idx1:closest_idx1 + ocp_N);
    else
        remaining_points1 = size(D1, 2) - closest_idx1 + 1;
        reference_points1 = D1(:, closest_idx1:end);
        additional_points1 = (ocp_N + 1) - remaining_points1;

        last_x1 = D1(1, end);
        last_y1 = D1(2, end);
        new_x1 = last_x1 - (1:additional_points1) * 0.1; % Assuming 0.1m per step
        new_y1 = last_y1 * ones(1, additional_points1);

        extended_points1 = [new_x1; new_y1];
        reference_points1 = [reference_points1, extended_points1];
    end
    
    % Reference points for car 2
    if closest_idx2 + ocp_N <= size(D2, 2)
        reference_points2 = D2(:, closest_idx2:closest_idx2 + ocp_N);
    else
        remaining_points2 = size(D2, 2) - closest_idx2 + 1;
        reference_points2 = D2(:, closest_idx2:end);
        additional_points2 = (ocp_N + 1) - remaining_points2;

        last_x2 = D2(1, end);
        last_y2 = D2(2, end);
        new_x2 = last_x2 + (1:additional_points2) * 0.1; % Assuming 0.1m per step
        new_y2 = last_y2 * ones(1, additional_points2);

        extended_points2 = [new_x2; new_y2];
        reference_points2 = [reference_points2, extended_points2];
    end

    % Create x_traj_init with the specified structure
    x_traj_init = [
        reference_points1; % x1, y1, ...
        testtheta1';       % theta1
        zeros(1, ocp_N + 1); % v1
        zeros(1, ocp_N + 1); % s1
        reference_points2; % x2, y2, ...
        testtheta2';       % theta2
        zeros(1, ocp_N + 1); % v2
        zeros(1, ocp_N + 1)  % s2
    ];

    % Check sizes
    S1 = size(x_traj_init, 1); % Number of rows
    S2 = size(x_traj_init, 2); % Number of columns

%     % Ensure that x_traj_init has enough rows
%     if S1 < 20
%         error('x_traj_init does not have enough rows. Current size: %d', S1);
%     end

    % Fill the parameter array with references and weights
    for jj = 0:ocp_N
        % Fill references for the first car
        p((jj) * (10 + 14) + 1:(jj) * (10 + 14) + 5) = x_traj_init(1:5, jj + 1); % Ref for car 1
        
        % Fill references for the second car
        p((jj) * (10 + 14) + 6:(jj) * (10 + 14) + 10) = x_traj_init(6:10, jj + 1); % Ref for car 2
        
        % Fill weights for the first car
        p((jj) * (10 + 14) + 11:(jj) * (10 + 14) + 15) = W_xu1(1:5); % Weights for car 1
        
        % Fill weights for the second car
        p((jj) * (10 + 14) + 16:(jj) * (10 + 14) + 20) = W_xu(1:5); % Weights for car 2
        
        % Fill weights for the control inputs
        p((jj) * (10 + 14) + 21:(jj) * (10 + 14) + 24) = [W_xu(6:7);W_xu1(6:7)]; % Control input weights (4 elements)
    end

    % Check if the size of p is correct
    assert(length(p) == 504, 'Parameter array must have 504 elements.');

    % Output parameter array
end

== matlab function Good_1PF_Template_Copy/MATLAB Function4 ==
  data: lbu output
function lbu = LBU
% Define lower bounds for control inputs
lbu_control = [-11.5; -1; -11.5; -1]; % Control inputs

% Determine how many times to repeat the control bounds
num_repeats = ceil(80 / length(lbu_control)); % Calculate how many times to repeat
lbu = repmat(lbu_control, num_repeats, 1); % Repeat to create a long enough array
lbu = lbu(1:80); % Truncate to exactly 80 elements

% Check size
assert(length(lbu) == 80, 'Lower bounds array must have 80 elements.');

end

== matlab function Good_1PF_Template_Copy/MATLAB Function5 ==
  data: ubu output
function ubu = UBU
% Define lower bounds for control inputs
ubu_control = [+11.5; 1; 11.5; 1]; % Control inputs

% Determine how many times to repeat the control bounds
num_repeats = ceil(80 / length(ubu_control)); % Calculate how many times to repeat
ubu = repmat(ubu_control, num_repeats, 1); % Repeat to create a long enough array
ubu = ubu(1:80); % Truncate to exactly 80 elements

% Check size
assert(length(ubu) == 80, 'Lower bounds array must have 80 elements.');

end

== matlab function Good_1PF_Template_Copy/PF_pred_trajectories/OCP_SOLVE_SFunction/MATLAB Function ==
  data: x0 input; p output; W_xu input; W_xu1 input; testtheta1 input; testtheta2 input; D1 input; D2 input; S1 output; S2 output
function [p, S1, S2] = OCP_prepare_parameters(x0, W_xu, W_xu1, testtheta1, testtheta2, D1, D2)
    nx = length(x0);
    nu = 4;
    ocp_N = 20; % Number of prediction steps
    % Initialize the parameter array
    p = zeros(504, 1); % 504 elements as per your structure

    % Prepare reference points
    current_state1 = x0(1:2); % Use the updated x0 for car 1
    current_state2 = x0(6:7); % Use the updated x0 for car 2
    
    closest_idx1 = findClosestPoint(current_state1, D1);
    closest_idx2 = findClosestPoint(current_state2, D2);
    
    % Reference points for car 1
    if closest_idx1 + ocp_N <= size(D1, 2)
        reference_points1 = D1(:, closest_idx1:closest_idx1 + ocp_N);
    else
        remaining_points1 = size(D1, 2) - closest_idx1 + 1;
        reference_points1 = D1(:, closest_idx1:end);
        additional_points1 = (ocp_N + 1) - remaining_points1;

        last_x1 = D1(1, end);
        last_y1 = D1(2, end);
        new_x1 = last_x1 - (1:additional_points1) * 0.1; % Assuming 0.1m per step
        new_y1 = last_y1 * ones(1, additional_points1);

        extended_points1 = [new_x1; new_y1];
        reference_points1 = [reference_points1, extended_points1];
    end
    
    % Reference points for car 2
    if closest_idx2 + ocp_N <= size(D2, 2)
        reference_points2 = D2(:, closest_idx2:closest_idx2 + ocp_N);
    else
        remaining_points2 = size(D2, 2) - closest_idx2 + 1;
        reference_points2 = D2(:, closest_idx2:end);
        additional_points2 = (ocp_N + 1) - remaining_points2;

        last_x2 = D2(1, end);
        last_y2 = D2(2, end);
        new_x2 = last_x2 + (1:additional_points2) * 0.1; % Assuming 0.1m per step
        new_y2 = last_y2 * ones(1, additional_points2);

        extended_points2 = [new_x2; new_y2];
        reference_points2 = [reference_points2, extended_points2];
    end

    % Create x_traj_init with the specified structure
    x_traj_init = [
        reference_points1; % x1, y1, ...
        testtheta1';       % theta1
        zeros(1, ocp_N + 1); % v1
        zeros(1, ocp_N + 1); % s1
        reference_points2; % x2, y2, ...
        testtheta2';       % theta2
        zeros(1, ocp_N + 1); % v2
        zeros(1, ocp_N + 1)  % s2
    ];

    % Check sizes
    S1 = size(x_traj_init, 1); % Number of rows
    S2 = size(x_traj_init, 2); % Number of columns

%     % Ensure that x_traj_init has enough rows
%     if S1 < 20
%         error('x_traj_init does not have enough rows. Current size: %d', S1);
%     end

    % Fill the parameter array with references and weights
    for jj = 0:ocp_N
        % Fill references for the first car
        p((jj) * (10 + 14) + 1:(jj) * (10 + 14) + 5) = x_traj_init(1:5, jj + 1); % Ref for car 1
        
        % Fill references for the second car
        p((jj) * (10 + 14) + 6:(jj) * (10 + 14) + 10) = x_traj_init(6:10, jj + 1); % Ref for car 2
        
        % Fill weights for the first car
        p((jj) * (10 + 14) + 11:(jj) * (10 + 14) + 15) = W_xu1(1:5); % Weights for car 1
        
        % Fill weights for the second car
        p((jj) * (10 + 14) + 16:(jj) * (10 + 14) + 20) = W_xu(1:5); % Weights for car 2
        
        % Fill weights for the control inputs
        p((jj) * (10 + 14) + 21:(jj) * (10 + 14) + 24) = [W_xu(6:7);W_xu1(6:7)]; % Control input weights (4 elements)
    end

    % Check if the size of p is correct
    assert(length(p) == 504, 'Parameter array must have 504 elements.');

    % Output parameter array
end

== matlab function Good_1PF_Template_Copy/PF_pred_trajectories/OCP_SOLVE_SFunction/MATLAB Function1 ==
  data: lbu output
function lbu = LBU
% Define lower bounds for control inputs
lbu_control = [-11.5; -1; -11.5; -1]; % Control inputs

% Determine how many times to repeat the control bounds
num_repeats = ceil(80 / length(lbu_control)); % Calculate how many times to repeat
lbu = repmat(lbu_control, num_repeats, 1); % Repeat to create a long enough array
lbu = lbu(1:80); % Truncate to exactly 80 elements

% Check size
assert(length(lbu) == 80, 'Lower bounds array must have 80 elements.');

end

== matlab function Good_1PF_Template_Copy/PF_pred_trajectories/OCP_SOLVE_SFunction/MATLAB Function2 ==
  data: ubu output
function ubu = UBU
% Define lower bounds for control inputs
ubu_control = [+11.5; 1; 11.5; 1]; % Control inputs

% Determine how many times to repeat the control bounds
num_repeats = ceil(80 / length(ubu_control)); % Calculate how many times to repeat
ubu = repmat(ubu_control, num_repeats, 1); % Repeat to create a long enough array
ubu = ubu(1:80); % Truncate to exactly 80 elements

% Check size
assert(length(ubu) == 80, 'Lower bounds array must have 80 elements.');

end

== matlab function Good_1PF_Template_Copy/PF_pred_trajectories/MATLAB Function ==
  data: u input; Y output size=[14,num_particles]; i input
function Y = fcn(u, i)
    persistent Y_storage; % Declare Y_storage as a persistent variable

    if isempty(Y_storage) % Initialize on the first call
        Y_storage = []; % Initialize as an empty array
    end

    if i == 1
        Y_storage = u; % Assign the first input directly
    else
        Y_storage = [Y_storage u]; % Concatenate the new input
    end

    Y = Y_storage; % Output the accumulated results
end
